simulink model "Preview_point_calculate_by_arc"  (R2021a)
settings: configuration reference "AION_IDS_Speedgoat" (kept outside this file)
libraries: simulink x1
settings Model: DataDictionary=Preview_Point_Calculate_By_Arc.sldd  Creator=xinrui  LastModifiedBy=Administrator
settings ConfigSetRef: SourceName=AION_IDS_Speedgoat

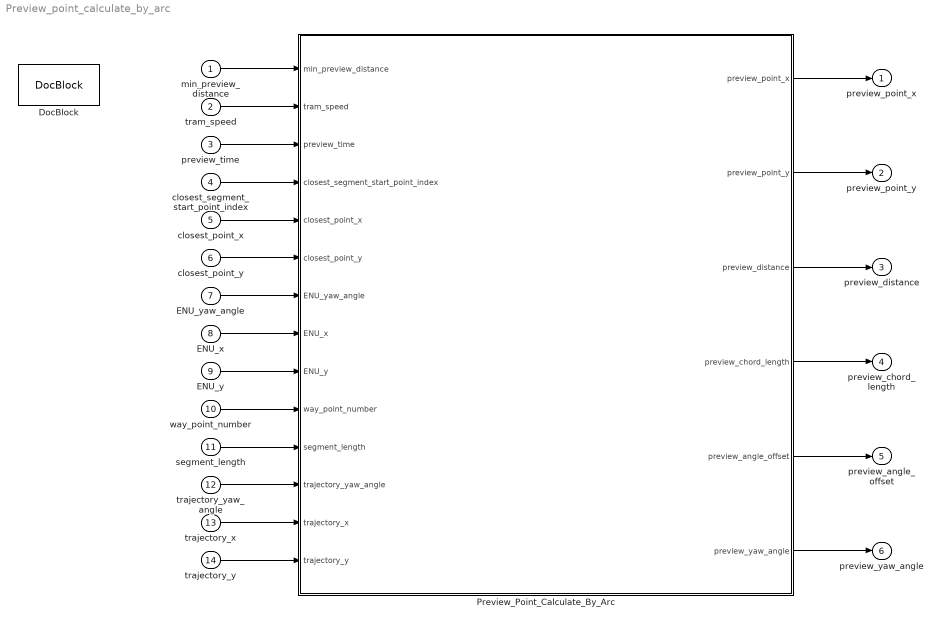
== system Preview_point_calculate_by_arc ==
  min_preview_distance : Inport  OutDataTypeStr=double  PortDimensions=1
  tram_speed : Inport  Port=2  OutDataTypeStr=double  PortDimensions=1
  preview_time : Inport  Port=3  OutDataTypeStr=double  PortDimensions=1
  closest_segment_start_point_index : Inport  Port=4  OutDataTypeStr=double  PortDimensions=1
  closest_point_x : Inport  Port=5  OutDataTypeStr=double  PortDimensions=1
  closest_point_y : Inport  Port=6  OutDataTypeStr=double  PortDimensions=1
  ENU_yaw_angle : Inport  Port=7  OutDataTypeStr=double  PortDimensions=1
  ENU_x : Inport  Port=8  OutDataTypeStr=double  PortDimensions=1
  ENU_y : Inport  Port=9  OutDataTypeStr=double  PortDimensions=1
  way_point_number : Inport  Port=10  OutDataTypeStr=double  PortDimensions=1
  segment_length : Inport  Port=11  OutDataTypeStr=double
  trajectory_yaw_angle : Inport  Port=12  OutDataTypeStr=double
  trajectory_x : Inport  Port=13  OutDataTypeStr=double
  trajectory_y : Inport  Port=14  OutDataTypeStr=double
  DocBlock : simulink/Model-Wide Utilities/DocBlock  DocumentType=HTML  mask(DocBlock){}
      mask Display:
      | plot([.8 0 0 1 1 .8 .8 1],[1 1 0 0 .8 1 .8 .8]);
      | text(.5,.6,'CHANGELOG','horizontalalignment','center');
      | text(.95,.05,get_param(gcb,'DocumentType'),'verticalalignment','bottom','horizontalalignment','right');
  Preview_Point_Calculate_By_Arc : MATLAB Function  TreatAsAtomicUnit=on
  preview_point_x : Outport  OutDataTypeStr=double  PortDimensions=1
  preview_point_y : Outport  Port=2  OutDataTypeStr=double  PortDimensions=1
  preview_distance : Outport  Port=3  OutDataTypeStr=double  PortDimensions=1
  preview_chord_length : Outport  Port=4  OutDataTypeStr=double  PortDimensions=1
  preview_angle_offset : Outport  Port=5  OutDataTypeStr=double  PortDimensions=1
  preview_yaw_angle : Outport  Port=6  OutDataTypeStr=double  PortDimensions=1
  wires:
  min_preview_distance/1 -> Preview_Point_Calculate_By_Arc/1(min_preview_distance)
  tram_speed/1 -> Preview_Point_Calculate_By_Arc/2(tram_speed)
  preview_time/1 -> Preview_Point_Calculate_By_Arc/3(preview_time)
  closest_segment_start_point_index/1 -> Preview_Point_Calculate_By_Arc/4(closest_segment_start_point_index)
  closest_point_x/1 -> Preview_Point_Calculate_By_Arc/5(closest_point_x)
  closest_point_y/1 -> Preview_Point_Calculate_By_Arc/6(closest_point_y)
  ENU_yaw_angle/1 -> Preview_Point_Calculate_By_Arc/7(ENU_yaw_angle)
  ENU_x/1 -> Preview_Point_Calculate_By_Arc/8(ENU_x)
  ENU_y/1 -> Preview_Point_Calculate_By_Arc/9(ENU_y)
  way_point_number/1 -> Preview_Point_Calculate_By_Arc/10(way_point_number)
  segment_length/1 -> Preview_Point_Calculate_By_Arc/11(segment_length)
  trajectory_yaw_angle/1 -> Preview_Point_Calculate_By_Arc/12(trajectory_yaw_angle)
  trajectory_x/1 -> Preview_Point_Calculate_By_Arc/13(trajectory_x)
  trajectory_y/1 -> Preview_Point_Calculate_By_Arc/14(trajectory_y)
  Preview_Point_Calculate_By_Arc/1(preview_point_x) -> preview_point_x/1
  Preview_Point_Calculate_By_Arc/2(preview_point_y) -> preview_point_y/1
  Preview_Point_Calculate_By_Arc/3(preview_distance) -> preview_distance/1
  Preview_Point_Calculate_By_Arc/4(preview_chord_length) -> preview_chord_length/1
  Preview_Point_Calculate_By_Arc/5(preview_angle_offset) -> preview_angle_offset/1
  Preview_Point_Calculate_By_Arc/6(preview_yaw_angle) -> preview_yaw_angle/1

== matlab function Preview_point_calculate_by_arc/Preview_Point_Calculate_By_Arc ==
  data: min_preview_distance input double size=1; tram_speed input double size=1; preview_point_x output double size=1; preview_time input double size=1; closest_segment_start_point_index input double size=1; closest_point_x input double size=1; preview_point_y output double size=1; preview_distance output double size=1; preview_chord_length output double size=1; closest_point_y input double size=1; ENU_yaw_angle input double size=1; ENU_x input double size=1; ENU_y input double size=1; preview_angle_offset output double size=1; way_point_number input double size=1; segment_length input double size=MAX_TRAJECTORY_WAY_POINT_NUMBER; trajectory_yaw_angle input double size=MAX_TRAJECTORY_WAY_POINT_NUMBER; trajectory_x input double size=MAX_TRAJECTORY_WAY_POINT_NUMBER; trajectory_y input double size=MAX_TRAJECTORY_WAY_POINT_NUMBER; ZERO_SPEED_THRESHOLD parameter double size=1; preview_yaw_angle output double size=1
% 通过弧长求参考轨迹上的预瞄点
function [preview_point_x, preview_point_y, preview_distance, preview_chord_length, ...
    preview_angle_offset, preview_yaw_angle] = Preview_point_calculate_by_arc(...
    min_preview_distance, tram_speed, preview_time, closest_segment_start_point_index, ...
    closest_point_x, closest_point_y, ENU_yaw_angle, ENU_x, ENU_y, way_point_number, ...
    segment_length, trajectory_yaw_angle, trajectory_x, trajectory_y, ZERO_SPEED_THRESHOLD)
%   1.输入参数：
%       (1)fixed_preview_distance               固定预瞄距离，m
%       (2)tram_speed                           整车车速，m/s
%       (3)preview_time                         预瞄时间，s
%       (4)closest_segment_start_point_index    最近路点线段起始点索引
%       (5)closest_point_x                      最近点x坐标，m
%       (6)closest_point_y                      最近点y坐标，m
%       (7)ENU_yaw_angle                        当前车辆在东北天坐标系下的横摆角，deg
%       (8)ENU_x                                当前车辆在东北天坐标系下的x坐标，m
%       (9)ENU_y                                当前车辆在东北天坐标系下的y坐标，m
%       (10)way_point_number                    局部路径路点个数
%       (11)segment_length                      路点间隔长度，m
%       (12)trajectory_yaw_angle                局部路径横摆角数组，有效数据数量为way_point_number
%       (13)trajectory_x                        局部路径x坐标数组，有效数据数量为way_point_number
%       (14)trajectory_y                        局部路径y坐标数组，有效数据数量为way_point_number
%   2.输出参数：
%       (1)preview_point_x                      预瞄点x坐标，m
%       (2)preview_point_y                      预瞄点y坐标，m
%       (3)preview_distance                     预瞄距离，m
%       (4)preview_chord_length                 预瞄弦长，m
%       (5)preview_angle_offset                 预瞄点处角度偏差，deg
%       (6)preview_yaw_angle                    预瞄点角度，deg

%% 静态变量声明及初始化
% 上周期预瞄点x坐标
persistent preview_point_x_previous;
if isempty(preview_point_x_previous)
   preview_point_x_previous = closest_point_x;
end

% 上周期预瞄点y坐标
persistent preview_point_y_previous;
if isempty(preview_point_y_previous)
   preview_point_y_previous = closest_point_y;
end

% 上周期预瞄点横摆角
persistent preview_yaw_angle_previous;
if isempty(preview_yaw_angle_previous)
   preview_yaw_angle_previous = 0;
end

%% 初始化
preview_point_valid               = false;   % 预瞄点有效标志，在循环中搜索到了则置为true
pass_previous_point_valid         = false;   % 通过上周期预瞄点有效标志，在循环中检测到了上周期预瞄点处于遍历线段的起点和终点之间则置为true

%% 求预瞄距离
% 低速用固定预瞄距离，高速用vt
preview_distance = max(tram_speed * preview_time, min_preview_distance);

%% 求预瞄弧长
% 计算最近点到本周期最近线段结束点的距离
distance = sqrt((closest_point_x - trajectory_x(closest_segment_start_point_index + 1)) ^ 2 + (...
    closest_point_y - trajectory_y(closest_segment_start_point_index + 1)) ^ 2);

% 从本周期最近线段结束点开始逐个路点循环搜索预瞄点
index = closest_segment_start_point_index + 1;
while preview_distance > distance && way_point_number > index
    % 切换下一个路点
    index = index + 1;
    
    % 弧长累加
    distance = distance + segment_length(index);
    
    % 向量投影法判断遍历路点是否经过上周期预瞄点
    [~, ~, projection_rate] = Vector_projection_get_closest_point_m(...
        preview_point_x_previous, preview_point_y_previous, ...
        trajectory_x(index - 1), trajectory_y(index - 1), ...
        trajectory_x(index), trajectory_y(index));
    if 1 >= projection_rate
        pass_previous_point_valid = true;
    end
end

% 预瞄线段结束点索引赋值
preview_segment_end_point_index = index;

% 当最近点到遍历路点的弧长距离大于预瞄距离时，可确定预瞄点
if way_point_number > preview_segment_end_point_index
    preview_point_valid = true;
end

%% 根据索引所处范围区间确定预瞄点及预瞄点处横摆角
if false == pass_previous_point_valid && ZERO_SPEED_THRESHOLD < tram_speed
    % 车辆在运动过程中预瞄点不后退，当标志位为false时，说明搜索没有经过上周期预瞄点，
    % 直接使用上周期预瞄点作为本周期预瞄点，确保预瞄点不后退
    preview_point_x = preview_point_x_previous;
    preview_point_y = preview_point_y_previous;
    preview_yaw_angle = preview_yaw_angle_previous;
elseif false == preview_point_valid
    % 到达参考路径终点后，使用终点作为本周期预瞄点
    preview_point_x = trajectory_x(way_point_number);
    preview_point_y = trajectory_y(way_point_number);
    preview_yaw_angle = trajectory_yaw_angle(way_point_number);
else
    % 通过线性插值求解本周期预瞄点
    delta_length = distance - preview_distance;
    preview_point_x = trajectory_x(preview_segment_end_point_index) - (delta_length / ...
        segment_length(preview_segment_end_point_index)) * (...
        trajectory_x(preview_segment_end_point_index) - ...
        trajectory_x(preview_segment_end_point_index - 1));
    preview_point_y = trajectory_y(preview_segment_end_point_index) - (delta_length / ...
        segment_length(preview_segment_end_point_index)) * (...
        trajectory_y(preview_segment_end_point_index) - ...
        trajectory_y(preview_segment_end_point_index - 1));
    preview_yaw_angle = trajectory_yaw_angle(preview_segment_end_point_index);
end

%% 求预瞄弦长
preview_chord_length = sqrt((preview_point_x - ENU_x) ^ 2 + (...
    preview_point_y - ENU_y) ^ 2);

%% 求预瞄点处角度偏差
% 对角度偏差加540再对360取模，最后减180，可确保输出的角度偏差在-180~180范围内
preview_angle_offset = mod(preview_yaw_angle - ENU_yaw_angle + 540, 360) - 180;

%% 相邻周期数据更新
preview_point_x_previous = preview_point_x;
preview_point_y_previous = preview_point_y;
preview_yaw_angle_previous = preview_yaw_angle;

end
